simulink model "DETUMBLE_POINTING"  (R2025b)
settings: Solver=ode45  StartTime=0.0  StopTime=5  RelTol=1e-3
values from neighbouring files (symbols this model uses):
  J = 0.002    [SIMULINK_Detumbling_Init.m]
  Jw = 1e-4    (= 0.0001)    [SIMULINK_Detumbling_Init.m]
  Kd = 0.01    [SIMULINK_Detumbling_Init.m]
  Kd_detumble = 0.03    [SIMULINK_Detumbling_Init.m]
  Kp = 0.02    [SIMULINK_Detumbling_Init.m]
  omega0 = deg2rad(8)    [SIMULINK_Detumbling_Init.m]
  omega_high = deg2rad(0.7)    [SIMULINK_Detumbling_Init.m]
  omega_low = deg2rad(0.3)    [SIMULINK_Detumbling_Init.m]
  omega_w0 = 0    [SIMULINK_Detumbling_Init.m]
  theta0 = deg2rad(15)    [SIMULINK_Detumbling_Init.m]
  theta_ref = deg2rad(theta_ref_deg)    [SIMULINK_Detumbling_Init.m]
settings Model: Creator=bbtp  LastModifiedBy=bbtp
settings SolverCC: ZeroCrossAlgorithm=Adaptive
settings DebuggingCC: IgnoredZcDiagnostic=none

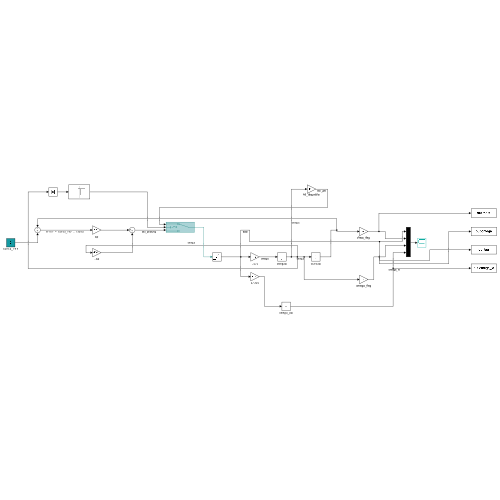
[thumbnail: Simulink's stored preview of the top-level diagram]
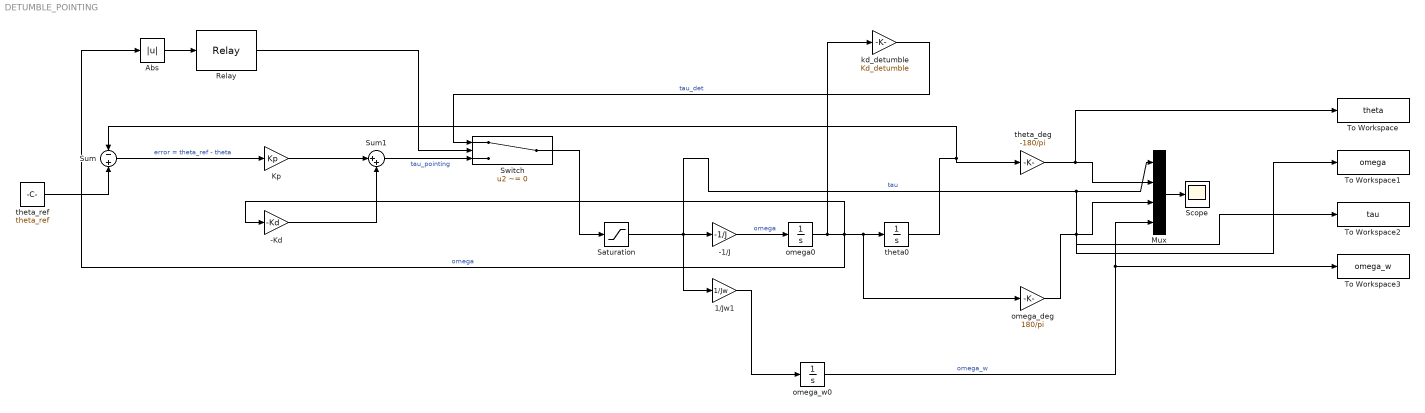
== system DETUMBLE_POINTING ==
  -1/J : Gain  Gain=-1/J
  -Kd : Gain  Gain=-Kd
  1/Jw1 : Gain  Gain=1/Jw
  Abs : Abs  SaturateOnIntegerOverflow=off
  Kp : Gain  Gain=Kp
  Mux : Mux
  Relay : Relay  OnSwitchValue=omega_high  OffSwitchValue=omega_low
  Saturation : Saturate
  Scope : Scope
      settings: ActiveDisplayYMinimum=-411567.73029706057  ActiveDisplayYMaximum=343540.60888628056
  Sum : Sum  Inputs=-+
  Sum1 : Sum  Inputs=|++
  Switch : Switch  Criteria=u2 ~= 0  SaturateOnIntegerOverflow=off  InputSameDT=off
  To Workspace : ToWorkspace  VariableName=theta  SaveFormat=Timeseries  SampleTime=-1
  To Workspace1 : ToWorkspace  VariableName=omega  SaveFormat=Timeseries  SampleTime=-1
  To Workspace2 : ToWorkspace  VariableName=tau  SaveFormat=Timeseries  SampleTime=-1
  To Workspace3 : ToWorkspace  VariableName=omega_w  SaveFormat=Timeseries  SampleTime=-1
  kd_detumble : Gain  Gain=Kd_detumble
  omega0 : Integrator  InitialCondition=omega0
  omega_deg : Gain  Gain=180/pi
  omega_w0 : Integrator  InitialCondition=omega_w0
  theta0 : Integrator  InitialCondition=-theta0
  theta_deg : Gain  Gain=-180/pi
  theta_ref : Constant  Value=theta_ref
  wires:
  Mux/1 -> Scope/1
  -Kd/1 -> Sum1/2
  theta0/1 -> Sum/1, theta_deg/1
  omega_deg/1 -> To Workspace1/1, Mux/3
  theta_ref/1 -> Sum/2
  theta_deg/1 -> To Workspace/1, Mux/2
  Kp/1 -> Sum1/1
  omega0/1 -> kd_detumble/1, Abs/1, -Kd/1, omega_deg/1, theta0/1  "omega"
  Saturation/1 -> 1/Jw1/1, To Workspace2/1, Mux/1, -1/J/1  "tau"
  Sum/1 -> Kp/1  "error = theta_ref - theta"
  Switch/1 -> Saturation/1
  kd_detumble/1 -> Switch/1  "tau_det"
  Sum1/1 -> Switch/3  "tau_pointing"
  Relay/1 -> Switch/2
  -1/J/1 -> omega0/1  "omega"
  1/Jw1/1 -> omega_w0/1
  omega_w0/1 -> To Workspace3/1, Mux/4  "omega_w"
  Abs/1 -> Relay/1
